simulink model "feedback_control"  (R2016a)
settings: Solver=FixedStepDiscrete  StartTime=0.0  StopTime=inf  FixedStep=T_sample_control  RelTol=1e-3
undefined symbols (not defined in the file): T_sample_control
settings Model: ModifiedByFormat=The MathWorks Inc.  Creator=The MathWorks, Inc.  LastModifiedBy=The MathWorks Inc.
settings DataIOCC: SaveFormat=Array
settings OptimizationCC: DefaultParameterBehavior=Inlined  InlineInvariantSignals=on  PassReuseOutputArgsThreshold=0  ExpressionDepthLimit=2147483647  EfficientFloat2IntCast=on
settings DebuggingCC: SolverPrmCheckMsg=warning  FcnCallInpInsideContextMsg=EnableAllAsWarning  UniqueDataStoreMsg=error  RootOutportRequireBusObject=error  AssertControl=DisableAll  AllowSymbolicDim=off  StateNameClashWarn=warning  StrictBusMsg=ErrorOnBusTreatedAsVector
settings HardwareCC: ProdBitPerPointer=32  ProdLargestAtomicInteger=Long  ProdWordSize=32  ProdHWDeviceType=ARM Compatible->ARM 7
settings ModelReferenceCC: PropagateSignalLabelsOutOfModel=off
settings RTWCC: SystemTargetFile=NIVeriStand_Linux_ARM_32.tlc  TemplateMakefile=NIVeriStand_Linux_ARM_32.tmf  Description=NI Linux Real-Time ARM (32-bit) Target  GenerateReport=on
settings STFCustomTargetCC: MatFileLogging=on  MATLABClassNameForMDSCustomization=Simulink.SoftwareTarget.TargetSpecificTriggerConfigurationBase  SystemTargetFile=NIVeriStand_Linux_ARM_32.tlc
settings ConfigComp: CovModelRefEnable=Off  CovSFcnEnable=off

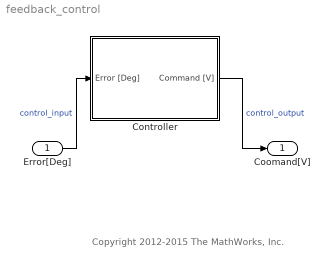
== system feedback_control ==
  note: Copyright 2012-2015 The MathWorks, Inc.
  Error[Deg] : Inport  OutDataTypeStr=double  PortDimensions=1  SampleTime=T_sample_control
  Controller : Subsystem
  Coomand[V] : Outport  OutDataTypeStr=double  PortDimensions=1  SampleTime=T_sample_control
  wires:
  Error[Deg]/1 -> Controller/1(Error [Deg])  "control_input"
  Controller/1(Command [V]) -> Coomand[V]/1  "control_output"

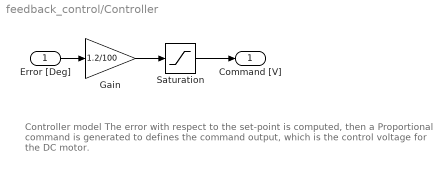
== system feedback_control/Controller ==
  note: Controller model
      | The error with respect to the set-point is computed, then a Proportional command
      | is generated to defines the command output, which is the control voltage for the DC motor.
  Error [Deg] : Inport
  Gain : Gain  Gain=1.2/100
  Saturation : Saturate  UpperLimit=1  LowerLimit=-1
  Command [V] : Outport
  wires:
  Gain/1 -> Saturation/1
  Error [Deg]/1 -> Gain/1
  Saturation/1 -> Command [V]/1
